simulink model "case2_brad_WB"  (Simulink 7.7)
settings: Solver=FixedStepDiscrete  StartTime=0.0  StopTime=Inf  RelTol=1e-3
undefined symbols (not defined in the file): node_param, path_param
libraries: SimpleModeling x38
settings Model: Creator=iris  LastModifiedBy=iris

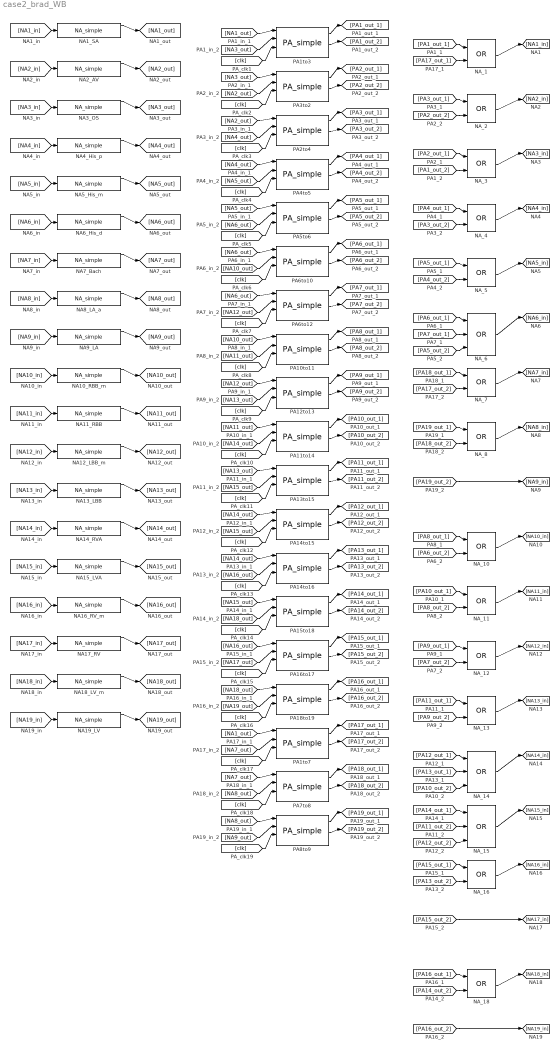
== system case2_brad_WB ==
  NA10_RBB_m : SimpleModeling/NA_simple  SystemSampleTime=-1  TERP_defs=node_param(10,2)  TRRP_def=node_param(10,4)  Trest_def=node_param(10,6)  TERP_s=node_param(10,1)  TRRP_s=node_param(10,3)  Trest_s=node_param(10,5)  Terp_min=node_param(10,7)  Terp_max=node_param(10,8)
  NA11_RBB : SimpleModeling/NA_simple  SystemSampleTime=-1  TERP_defs=node_param(11,2)  TRRP_def=node_param(11,4)  Trest_def=node_param(11,6)  TERP_s=node_param(11,1)  TRRP_s=node_param(11,3)  Trest_s=node_param(11,5)  Terp_min=node_param(11,7)  Terp_max=node_param(11,8)
  NA12_LBB_m : SimpleModeling/NA_simple  SystemSampleTime=-1  TERP_defs=node_param(12,2)  TRRP_def=node_param(12,4)  Trest_def=node_param(12,6)  TERP_s=node_param(12,1)  TRRP_s=node_param(12,3)  Trest_s=node_param(12,5)  Terp_min=node_param(12,7)  Terp_max=node_param(12,8)
  NA13_LBB : SimpleModeling/NA_simple  SystemSampleTime=-1  TERP_defs=node_param(13,2)  TRRP_def=node_param(13,4)  Trest_def=node_param(13,6)  TERP_s=node_param(13,1)  TRRP_s=node_param(13,3)  Trest_s=node_param(13,5)  Terp_min=node_param(13,7)  Terp_max=node_param(13,8)
  NA14_RVA : SimpleModeling/NA_simple  SystemSampleTime=-1  TERP_defs=node_param(14,2)  TRRP_def=node_param(14,4)  Trest_def=node_param(14,6)  TERP_s=node_param(14,1)  TRRP_s=node_param(14,3)  Trest_s=node_param(14,5)  Terp_min=node_param(14,7)  Terp_max=node_param(14,8)
  NA15_LVA : SimpleModeling/NA_simple  SystemSampleTime=-1  TERP_defs=node_param(15,2)  TRRP_def=node_param(15,4)  Trest_def=node_param(15,6)  TERP_s=node_param(15,1)  TRRP_s=node_param(15,3)  Trest_s=node_param(15,5)  Terp_min=node_param(15,7)  Terp_max=node_param(15,8)
  NA16_RV_m : SimpleModeling/NA_simple  SystemSampleTime=-1  TERP_defs=node_param(16,2)  TRRP_def=node_param(16,4)  Trest_def=node_param(16,6)  TERP_s=node_param(16,1)  TRRP_s=node_param(16,3)  Trest_s=node_param(16,5)  Terp_min=node_param(16,7)  Terp_max=node_param(16,8)
  NA17_RV : SimpleModeling/NA_simple  SystemSampleTime=-1  TERP_defs=node_param(17,2)  TRRP_def=node_param(17,4)  Trest_def=node_param(17,6)  TERP_s=node_param(17,1)  TRRP_s=node_param(17,3)  Trest_s=node_param(17,5)  Terp_min=node_param(17,7)  Terp_max=node_param(17,8)
  NA18_LV_m : SimpleModeling/NA_simple  SystemSampleTime=-1  TERP_defs=node_param(18,2)  TRRP_def=node_param(18,4)  Trest_def=node_param(18,6)  TERP_s=node_param(18,1)  TRRP_s=node_param(18,3)  Trest_s=node_param(18,5)  Terp_min=node_param(18,7)  Terp_max=node_param(18,8)
  NA19_LV : SimpleModeling/NA_simple  SystemSampleTime=-1  TERP_defs=node_param(19,2)  TRRP_def=node_param(19,4)  Trest_def=node_param(19,6)  TERP_s=node_param(19,1)  TRRP_s=node_param(19,3)  Trest_s=node_param(19,5)  Terp_min=node_param(19,7)  Terp_max=node_param(19,8)
  NA1_SA : SimpleModeling/NA_simple  SystemSampleTime=-1  TERP_defs=node_param(1,2)  TRRP_def=node_param(1,4)  Trest_def=node_param(1,6)  TERP_s=node_param(1,1)  TRRP_s=node_param(1,3)  Trest_s=node_param(1,5)  Terp_min=node_param(1,7)  Terp_max=node_param(1,8)
  NA2_AV : SimpleModeling/NA_simple  SystemSampleTime=-1  TERP_defs=node_param(2,2)  TRRP_def=node_param(2,4)  Trest_def=node_param(2,6)  TERP_s=node_param(2,1)  TRRP_s=node_param(2,3)  Trest_s=node_param(2,5)  Terp_min=node_param(2,7)  Terp_max=node_param(2,8)
  NA3_OS : SimpleModeling/NA_simple  SystemSampleTime=-1  TERP_defs=node_param(3,2)  TRRP_def=node_param(3,4)  Trest_def=node_param(3,6)  TERP_s=node_param(3,1)  TRRP_s=node_param(3,3)  Trest_s=node_param(3,5)  Terp_min=node_param(3,7)  Terp_max=node_param(3,8)
  NA4_His_p : SimpleModeling/NA_simple  SystemSampleTime=-1  TERP_defs=node_param(4,2)  TRRP_def=node_param(4,4)  Trest_def=node_param(4,6)  TERP_s=node_param(4,1)  TRRP_s=node_param(4,3)  Trest_s=node_param(4,5)  Terp_min=node_param(4,7)  Terp_max=node_param(4,8)
  NA5_His_m : SimpleModeling/NA_simple  SystemSampleTime=-1  TERP_defs=node_param(5,2)  TRRP_def=node_param(5,4)  Trest_def=node_param(5,6)  TERP_s=node_param(5,1)  TRRP_s=node_param(5,3)  Trest_s=node_param(5,5)  Terp_min=node_param(5,7)  Terp_max=node_param(5,8)
  NA6_His_d : SimpleModeling/NA_simple  SystemSampleTime=-1  TERP_defs=node_param(6,2)  TRRP_def=node_param(6,4)  Trest_def=node_param(6,6)  TERP_s=node_param(6,1)  TRRP_s=node_param(6,3)  Trest_s=node_param(6,5)  Terp_min=node_param(6,7)  Terp_max=node_param(6,8)
  NA7_Bach : SimpleModeling/NA_simple  SystemSampleTime=-1  TERP_defs=node_param(7,2)  TRRP_def=node_param(7,4)  Trest_def=node_param(7,6)  TERP_s=node_param(7,1)  TRRP_s=node_param(7,3)  Trest_s=node_param(7,5)  Terp_min=node_param(7,7)  Terp_max=node_param(7,8)
  NA8_LA_a : SimpleModeling/NA_simple  SystemSampleTime=-1  TERP_defs=node_param(8,2)  TRRP_def=node_param(8,4)  Trest_def=node_param(8,6)  TERP_s=node_param(8,1)  TRRP_s=node_param(8,3)  Trest_s=node_param(8,5)  Terp_min=node_param(8,7)  Terp_max=node_param(8,8)
  NA9_LA : SimpleModeling/NA_simple  SystemSampleTime=-1  TERP_defs=node_param(9,2)  TRRP_def=node_param(9,4)  Trest_def=node_param(9,6)  TERP_s=node_param(9,1)  TRRP_s=node_param(9,3)  Trest_s=node_param(9,5)  Terp_min=node_param(9,7)  Terp_max=node_param(9,8)
  NA_{1..5,7..8,10..13,16,18} (13 alike) : Logic  Operator=OR  AllPortsSameDT=off  OutDataTypeStr=boolean
  NA_14 : Logic  Operator=OR  Inputs=3  AllPortsSameDT=off  OutDataTypeStr=boolean
  NA_15 : Logic  Operator=OR  Inputs=3  AllPortsSameDT=off  OutDataTypeStr=boolean
  NA_6 : Logic  Operator=OR  Inputs=3  AllPortsSameDT=off  OutDataTypeStr=boolean
  PA10to11 : SimpleModeling/PA_simple  SystemSampleTime=-1  min_path_par=path_param(10,11,5)  bck_param=path_param(10,11,7)  forw_param=path_param(10,11,6)
  PA11to14 : SimpleModeling/PA_simple  SystemSampleTime=-1  min_path_par=path_param(11,14,5)  bck_param=path_param(11,14,7)  forw_param=path_param(11,14,6)
  PA12to13 : SimpleModeling/PA_simple  SystemSampleTime=-1  min_path_par=path_param(12,13,5)  bck_param=path_param(12,13,7)  forw_param=path_param(12,13,6)
  PA13to15 : SimpleModeling/PA_simple  SystemSampleTime=-1  min_path_par=path_param(13,15,5)  bck_param=path_param(13,15,7)  forw_param=path_param(13,15,6)
  PA14to15 : SimpleModeling/PA_simple  SystemSampleTime=-1  min_path_par=path_param(14,15,5)  bck_param=path_param(14,15,7)  forw_param=path_param(14,15,6)
  PA14to16 : SimpleModeling/PA_simple  SystemSampleTime=-1  min_path_par=path_param(14,16,5)  bck_param=path_param(14,16,7)  forw_param=path_param(14,16,6)
  PA15to18 : SimpleModeling/PA_simple  SystemSampleTime=-1  min_path_par=path_param(15,18,5)  bck_param=path_param(15,18,7)  forw_param=path_param(15,18,6)
  PA16to17 : SimpleModeling/PA_simple  SystemSampleTime=-1  min_path_par=path_param(16,17,5)  bck_param=path_param(16,17,7)  forw_param=path_param(16,17,6)
  PA18to19 : SimpleModeling/PA_simple  SystemSampleTime=-1  min_path_par=path_param(18,19,5)  bck_param=path_param(18,19,7)  forw_param=path_param(18,19,6)
  PA1to3 : SimpleModeling/PA_simple  SystemSampleTime=-1  min_path_par=path_param(1,3,5)  bck_param=path_param(1,3,7)  forw_param=path_param(1,3,6)
  PA1to7 : SimpleModeling/PA_simple  SystemSampleTime=-1  min_path_par=path_param(1,7,5)  bck_param=path_param(1,7,7)  forw_param=path_param(1,7,6)
  PA2to4 : SimpleModeling/PA_simple  SystemSampleTime=-1  min_path_par=path_param(2,4,5)  bck_param=path_param(2,4,7)  forw_param=path_param(2,4,6)
  PA3to2 : SimpleModeling/PA_simple  SystemSampleTime=-1  min_path_par=path_param(3,2,5)  bck_param=path_param(3,2,7)  forw_param=path_param(3,2,6)
  PA4to5 : SimpleModeling/PA_simple  SystemSampleTime=-1  min_path_par=path_param(4,5,5)  bck_param=path_param(4,5,7)  forw_param=path_param(4,5,6)
  PA5to6 : SimpleModeling/PA_simple  SystemSampleTime=-1  min_path_par=path_param(5,6,5)  bck_param=path_param(5,6,7)  forw_param=path_param(5,6,6)
  PA6to10 : SimpleModeling/PA_simple  SystemSampleTime=-1  min_path_par=path_param(6,10,5)  bck_param=path_param(6,10,7)  forw_param=path_param(6,10,6)
  PA6to12 : SimpleModeling/PA_simple  SystemSampleTime=-1  min_path_par=path_param(6,12,5)  bck_param=path_param(6,12,7)  forw_param=path_param(6,12,6)
  PA7to8 : SimpleModeling/PA_simple  SystemSampleTime=-1  min_path_par=path_param(7,8,5)  bck_param=path_param(7,8,7)  forw_param=path_param(7,8,6)
  PA8to9 : SimpleModeling/PA_simple  SystemSampleTime=-1  min_path_par=path_param(8,9,5)  bck_param=path_param(8,9,7)  forw_param=path_param(8,9,6)
  wires:
  NA1_SA/1 -> [NA1_out]
  [NA1_in] -> NA1_SA/1
  [PA1_out_1] -> NA_1/1
  [PA17_out_1] -> NA_1/2
  NA_1/1 -> [NA1_in]
  NA2_AV/1 -> [NA2_out]
  [NA2_in] -> NA2_AV/1
  [PA3_out_1] -> NA_2/1
  [PA2_out_2] -> NA_2/2
  NA_2/1 -> [NA2_in]
  NA3_OS/1 -> [NA3_out]
  [NA3_in] -> NA3_OS/1
  [PA2_out_1] -> NA_3/1
  [PA1_out_2] -> NA_3/2
  NA_3/1 -> [NA3_in]
  NA4_His_p/1 -> [NA4_out]
  [NA4_in] -> NA4_His_p/1
  [PA4_out_1] -> NA_4/1
  [PA3_out_2] -> NA_4/2
  NA_4/1 -> [NA4_in]
  NA5_His_m/1 -> [NA5_out]
  [NA5_in] -> NA5_His_m/1
  [PA5_out_1] -> NA_5/1
  [PA4_out_2] -> NA_5/2
  NA_5/1 -> [NA5_in]
  NA6_His_d/1 -> [NA6_out]
  [NA6_in] -> NA6_His_d/1
  [PA6_out_1] -> NA_6/1
  [PA7_out_1] -> NA_6/2
  [PA5_out_2] -> NA_6/3
  NA_6/1 -> [NA6_in]
  NA7_Bach/1 -> [NA7_out]
  [NA7_in] -> NA7_Bach/1
  [PA18_out_1] -> NA_7/1
  [PA17_out_2] -> NA_7/2
  NA_7/1 -> [NA7_in]
  NA8_LA_a/1 -> [NA8_out]
  [NA8_in] -> NA8_LA_a/1
  [PA19_out_1] -> NA_8/1
  [PA18_out_2] -> NA_8/2
  NA_8/1 -> [NA8_in]
  NA9_LA/1 -> [NA9_out]
  [NA9_in] -> NA9_LA/1
  [PA19_out_2] -> [NA9_in]
  NA10_RBB_m/1 -> [NA10_out]
  [NA10_in] -> NA10_RBB_m/1
  [PA8_out_1] -> NA_10/1
  [PA6_out_2] -> NA_10/2
  NA_10/1 -> [NA10_in]
  NA11_RBB/1 -> [NA11_out]
  [NA11_in] -> NA11_RBB/1
  [PA10_out_1] -> NA_11/1
  [PA8_out_2] -> NA_11/2
  NA_11/1 -> [NA11_in]
  NA12_LBB_m/1 -> [NA12_out]
  [NA12_in] -> NA12_LBB_m/1
  [PA9_out_1] -> NA_12/1
  [PA7_out_2] -> NA_12/2
  NA_12/1 -> [NA12_in]
  NA13_LBB/1 -> [NA13_out]
  [NA13_in] -> NA13_LBB/1
  [PA11_out_1] -> NA_13/1
  [PA9_out_2] -> NA_13/2
  NA_13/1 -> [NA13_in]
  NA14_RVA/1 -> [NA14_out]
  [NA14_in] -> NA14_RVA/1
  [PA12_out_1] -> NA_14/1
  [PA13_out_1] -> NA_14/2
  [PA10_out_2] -> NA_14/3
  NA_14/1 -> [NA14_in]
  NA15_LVA/1 -> [NA15_out]
  [NA15_in] -> NA15_LVA/1
  [PA14_out_1] -> NA_15/1
  [PA11_out_2] -> NA_15/2
  [PA12_out_2] -> NA_15/3
  NA_15/1 -> [NA15_in]
  NA16_RV_m/1 -> [NA16_out]
  [NA16_in] -> NA16_RV_m/1
  [PA15_out_1] -> NA_16/1
  [PA13_out_2] -> NA_16/2
  NA_16/1 -> [NA16_in]
  NA17_RV/1 -> [NA17_out]
  [NA17_in] -> NA17_RV/1
  [PA15_out_2] -> [NA17_in]
  NA18_LV_m/1 -> [NA18_out]
  [NA18_in] -> NA18_LV_m/1
  [PA16_out_1] -> NA_18/1
  [PA14_out_2] -> NA_18/2
  NA_18/1 -> [NA18_in]
  NA19_LV/1 -> [NA19_out]
  [NA19_in] -> NA19_LV/1
  [PA16_out_2] -> [NA19_in]
  PA1to3/1 -> [PA1_out_1]
  PA1to3/2 -> [PA1_out_2]
  [NA1_out] -> PA1to3/1
  [NA3_out] -> PA1to3/2
  [clk] -> PA1to3/3
  PA3to2/1 -> [PA2_out_1]
  PA3to2/2 -> [PA2_out_2]
  [NA3_out] -> PA3to2/1
  [NA2_out] -> PA3to2/2
  [clk] -> PA3to2/3
  PA2to4/1 -> [PA3_out_1]
  PA2to4/2 -> [PA3_out_2]
  [NA2_out] -> PA2to4/1
  [NA4_out] -> PA2to4/2
  [clk] -> PA2to4/3
  PA4to5/1 -> [PA4_out_1]
  PA4to5/2 -> [PA4_out_2]
  [NA4_out] -> PA4to5/1
  [NA5_out] -> PA4to5/2
  [clk] -> PA4to5/3
  PA5to6/1 -> [PA5_out_1]
  PA5to6/2 -> [PA5_out_2]
  [NA5_out] -> PA5to6/1
  [NA6_out] -> PA5to6/2
  [clk] -> PA5to6/3
  PA6to10/1 -> [PA6_out_1]
  PA6to10/2 -> [PA6_out_2]
  [NA6_out] -> PA6to10/1
  [NA10_out] -> PA6to10/2
  [clk] -> PA6to10/3
  PA6to12/1 -> [PA7_out_1]
  PA6to12/2 -> [PA7_out_2]
  [NA6_out] -> PA6to12/1
  [NA12_out] -> PA6to12/2
  [clk] -> PA6to12/3
  PA10to11/1 -> [PA8_out_1]
  PA10to11/2 -> [PA8_out_2]
  [NA10_out] -> PA10to11/1
  [NA11_out] -> PA10to11/2
  [clk] -> PA10to11/3
  PA12to13/1 -> [PA9_out_1]
  PA12to13/2 -> [PA9_out_2]
  [NA12_out] -> PA12to13/1
  [NA13_out] -> PA12to13/2
  [clk] -> PA12to13/3
  PA11to14/1 -> [PA10_out_1]
  PA11to14/2 -> [PA10_out_2]
  [NA11_out] -> PA11to14/1
  [NA14_out] -> PA11to14/2
  [clk] -> PA11to14/3
  PA13to15/1 -> [PA11_out_1]
  PA13to15/2 -> [PA11_out_2]
  [NA13_out] -> PA13to15/1
  [NA15_out] -> PA13to15/2
  [clk] -> PA13to15/3
  PA14to15/1 -> [PA12_out_1]
  PA14to15/2 -> [PA12_out_2]
  [NA14_out] -> PA14to15/1
  [NA15_out] -> PA14to15/2
  [clk] -> PA14to15/3
  PA14to16/1 -> [PA13_out_1]
  PA14to16/2 -> [PA13_out_2]
  [NA14_out] -> PA14to16/1
  [NA16_out] -> PA14to16/2
  [clk] -> PA14to16/3
  PA15to18/1 -> [PA14_out_1]
  PA15to18/2 -> [PA14_out_2]
  [NA15_out] -> PA15to18/1
  [NA18_out] -> PA15to18/2
  [clk] -> PA15to18/3
  PA16to17/1 -> [PA15_out_1]
  PA16to17/2 -> [PA15_out_2]
  [NA16_out] -> PA16to17/1
  [NA17_out] -> PA16to17/2
  [clk] -> PA16to17/3
  PA18to19/1 -> [PA16_out_1]
  PA18to19/2 -> [PA16_out_2]
  [NA18_out] -> PA18to19/1
  [NA19_out] -> PA18to19/2
  [clk] -> PA18to19/3
  PA1to7/1 -> [PA17_out_1]
  PA1to7/2 -> [PA17_out_2]
  [NA1_out] -> PA1to7/1
  [NA7_out] -> PA1to7/2
  [clk] -> PA1to7/3
  PA7to8/1 -> [PA18_out_1]
  PA7to8/2 -> [PA18_out_2]
  [NA7_out] -> PA7to8/1
  [NA8_out] -> PA7to8/2
  [clk] -> PA7to8/3
  PA8to9/1 -> [PA19_out_1]
  PA8to9/2 -> [PA19_out_2]
  [NA8_out] -> PA8to9/1
  [NA9_out] -> PA8to9/2
  [clk] -> PA8to9/3
